simulink model "etherCATmdl3"  (R2022a)
settings: Solver=FixedStepDiscrete  StartTime=0.0  StopTime=inf  RelTol=1e-3
PreLoadFcn:
  | Ts_IO133 = 0.001;
  | Ts_IO750 = 0.001;
InitFcn:
  | Ts_IO133 = 0.001
StopFcn:
  | if isfile(['sdi_view_',bdroot,'.mldatx'])
  |  Simulink.sdi.clearPreferences();
  |  Simulink.sdi.view();
  |  pause(3);
  |  Simulink.sdi.loadView(['sdi_view_',bdroot,]);
  | end
undefined symbols (not defined in the file or in its folder): AUS0, AUS1, C, CAN, FD, padding, Statuswort, Steuerwort
libraries: speedgoatlib_IO602 x9, slrealtimeutilitieslib x8, speedgoatlib_IO133 x5, canfdmsglib x4, canmsglib x4, speedgoatlib_IO750 x4, etargetslib x3, simulink x1
settings Model: SimulationMode=external  ExtModeEnableFloating=off  Creator=sandro.reichenbach  LastModifiedBy=muhammet.cingoez
settings SolverCC: ConcurrentTasks=on  PositivePriorityOrder=on
settings DataIOCC: LimitDataPoints=on  SaveFormat=StructureWithTime
settings OptimizationCC: BlockReduction=off  OptimizeBlockIOStorage=off
settings DebuggingCC: TasksWithSamePriorityMsg=none
settings HardwareCC: ProdBitPerLong=64  ProdLongLongMode=on  ProdHWDeviceType=Intel->x86-64 (Linux 64)
settings RTWCC: Description=Simulink Real-Time  SystemTargetFile=slrealtime.tlc  TemplateMakefile=slrealtime_default_tmf  RTWVerbose=off  Toolchain=Simulink Real-Time Toolchain  BuildConfiguration=Faster Runs  CodeExecutionProfiling=on  TargetLang=C++  DLArmComputeVersion=19.05

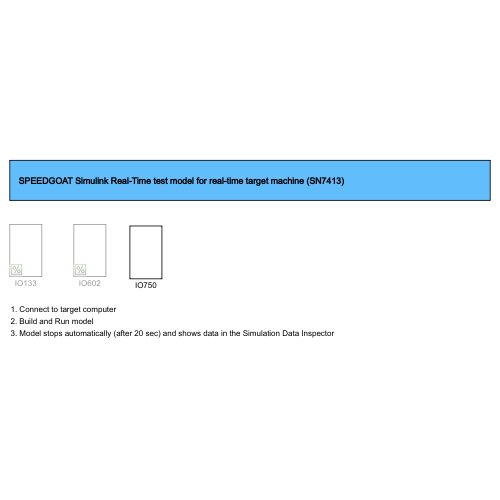
[thumbnail: Simulink's stored preview of the top-level diagram]
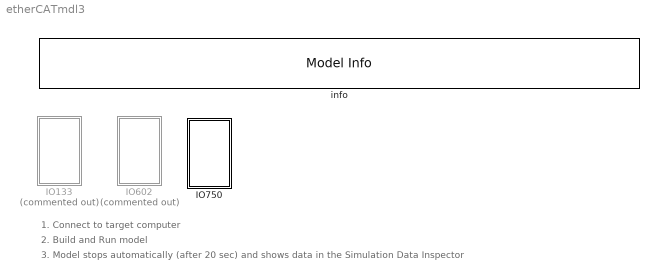
== system etherCATmdl3 ==
  note: 1. Connect to target computer
  note: 2. Build and Run model
  note: 3. Model stops automatically (after 20 sec) and shows data in the Simulation Data Inspector
  IO133 : Subsystem  Commented=on
  IO602 : Subsystem  Commented=on
  IO750 : Subsystem
  info : simulink/Model-Wide Utilities/Model Info  Frame=on  DisplayStringWithTags=SPEEDGOAT Simulink Real-Time test model for real-time target machine (SN7413)  HorizontalTextAlignment=Left  LeftAlignmentValue=0.02

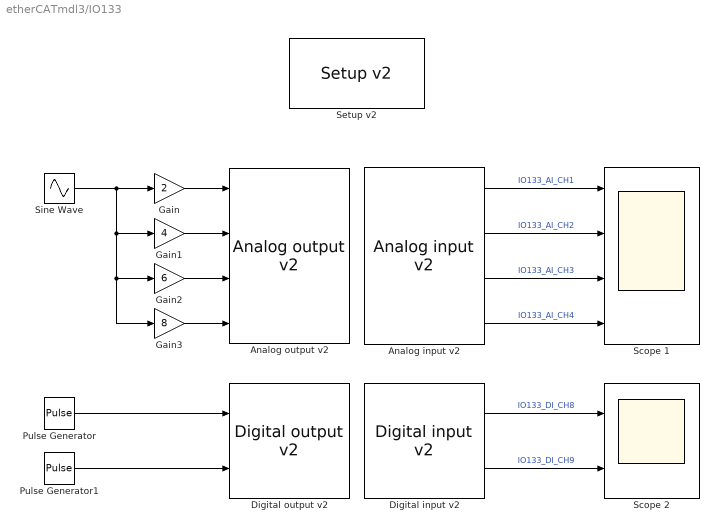
== system etherCATmdl3/IO133 ==
  "Analog input v2 " : speedgoatlib_IO133/Analog input v2   parModuleId=1  parSampleTime=Ts_IO133  parPciSlot=-1  parAdcChannels=[1 2 3 4]  parAdcVoltageRange=[2 2]  parAdcOversamplRate=[1 1]  parAdcContSampling=0  parAdcDmaEnable=0  parAdcActiveDmaDevices=[1 1]  parAdcFrameSize=100
      settings: SourceProductName=Simulink Real-Time: Speedgoat I/O Driver Library
  "Analog output v2 " : speedgoatlib_IO133/Analog output v2   parModuleId=1  parSampleTime=Ts_IO133  parPciSlot=-1  parDacChannels=[1 2 3 4]  parDacVoltageRange=[4 4 6 6 5 5 5 5]  parDacInitValues=[0 0 0 0]  parDacReset=[1 1 1 1]  parDacSyncOut=1  parDacDmaEnable=0  parDacActiveDmaDevices=[1 1]  parDacDmaLatency=2  parDacFrameSize=100
      settings: SourceProductName=Simulink Real-Time: Speedgoat I/O Driver Library
  "Digital input v2 " : speedgoatlib_IO133/Digital input v2   parModuleId=1  parSampleTime=Ts_IO133  parPciSlot=-1  parDiChannels=[8 9]
      settings: SourceProductName=Simulink Real-Time: Speedgoat I/O Driver Library
  "Digital output v2 " : speedgoatlib_IO133/Digital output v2   parModuleId=1  parSampleTime=Ts_IO133  parPciSlot=-1  parDoChannels=[1 2]  parDoInitValues=[0 0]  parDoReset=[1 1]
      settings: SourceProductName=Simulink Real-Time: Speedgoat I/O Driver Library
  Gain : Gain  Gain=2
  Gain1 : Gain  Gain=4
  Gain2 : Gain  Gain=6
  Gain3 : Gain  Gain=8
  Pulse Generator : DiscretePulseGenerator  Period=20  PulseWidth=5  SampleTime=-1
  Pulse Generator1 : DiscretePulseGenerator  Period=20  PulseWidth=10  SampleTime=-1
  Scope 1 : Scope  NumInputPorts=4
  Scope 2 : Scope  NumInputPorts=2
  "Setup v2 " : speedgoatlib_IO133/Setup v2   parPciSlot=-1  parModuleId=1  parInterModuleSync=None  parConvClockBaseRate=20MHz  parConvClock1Divider=20000  parConvClock2Divider=20000  parFrameTriggerEnable=off  parFrameTriggerDivider=10  parConvClock1BaseRate=1  parConvClock2BaseRate=1  parFrameTriggerClock=1  parAdcChannels=1:4  parAdcRange1=+-10V  parAdcRange2=+-10V  parAdcVoltageRange=[2 2]  parAdcOversampling1=None  parAdcOversampling2=None  parAdcOversamplRate=[1 1]  parAdcAutoCorrection=on  parAdcContSampling=off  parAdcDmaEnable=off  parAdcDmaClock=Clock 1  parAdcFrameSize_=100  parAdcSampleTime_=-1  parAdcActiveDmaDevices=[1 1]  parAdcFrameTriggerEnable=0  parAdcFrameSize=100  parAdcSampleTime=0.1  parDacChannels=1:4  parDacInitValues=0  parDacReset=1  parDacRange1=+-5V  parDacRange2=+-5V  parDacRange3=+-10.8V  parDacRange4=+-10.8V  parDacRange5=+-10V  parDacRange6=+-10V  parDacRange7=+-10V  parDacRange8=+-10V  parDacVoltageRange=[4 4 6 6 5 5 5 5]  parDacAutoCorrection=on  parDacSyncOut=on  parDacDmaEnable=off  parDacDmaLatency=Until next frame  parDacDmaClock=Clock 1  parDacFrameSize_=100  parDacSampleTime_=-1  parDacActiveDmaDevices=[1 1]  parDacFrameTriggerEnable=0  parDacFrameSize=100  parDacSampleTime=0.1  parDoChannels=1:2  parDoInitValues=0  parDoReset=1  parDiChannels=8:9  parDiDebounceEnable=off  parDiDebounceTime=0  parDiDebounceValue=0  parDioPullRefFront=Pull-up 3.3V  parDioPullRefRear=Floating
      settings: SourceProductName=Simulink Real-Time: Speedgoat I/O Driver Library
  Sine Wave : Sin  Frequency=50  SampleTime=0
  wires:
  Pulse Generator/1 -> "Digital output v2 "/1
  Gain1/1 -> "Analog output v2 "/2
  Gain/1 -> "Analog output v2 "/1
  Gain3/1 -> "Analog output v2 "/4
  Gain2/1 -> "Analog output v2 "/3
  Sine Wave/1 -> Gain/1, Gain1/1, Gain2/1, Gain3/1
  Pulse Generator1/1 -> "Digital output v2 "/2
  "Analog input v2 "/1 -> Scope 1/1  "IO133_AI_CH1"
  "Analog input v2 "/2 -> Scope 1/2  "IO133_AI_CH2"
  "Analog input v2 "/3 -> Scope 1/3  "IO133_AI_CH3"
  "Analog input v2 "/4 -> Scope 1/4  "IO133_AI_CH4"
  "Digital input v2 "/1 -> Scope 2/1  "IO133_DI_CH8"
  "Digital input v2 "/2 -> Scope 2/2  "IO133_DI_CH9"

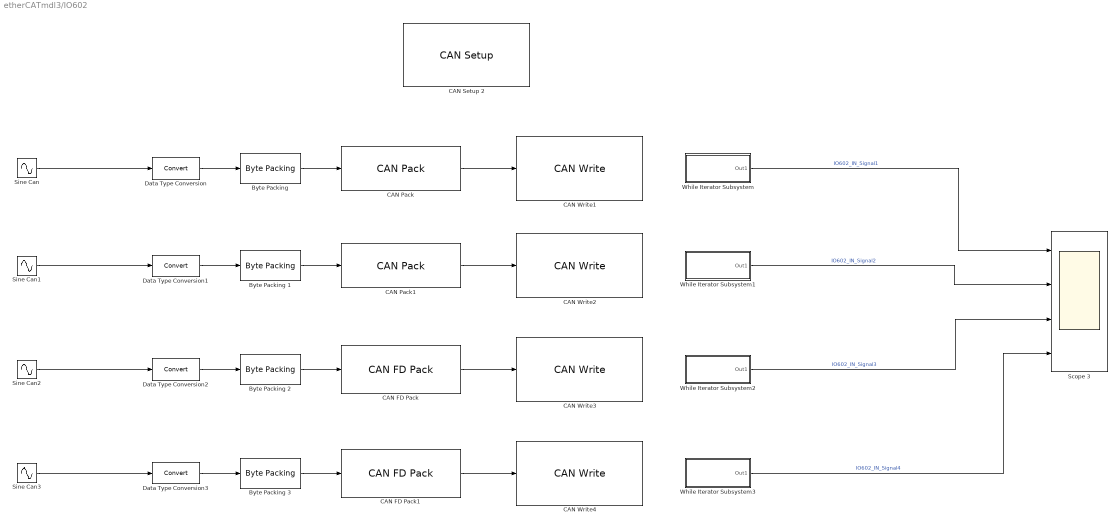
== system etherCATmdl3/IO602 ==
  Byte Packing {,1..3} (4 alike) : slrealtimeutilitieslib/Byte Packing  MaskPackedDataType=uint8  MaskUnpackedDataTypes={'single'}  MaskAlignment=1
  CAN FD Pack : canfdmsglib/CAN FD Pack  MsgList=(none)  MsgName=Msg  ProtocolMode=CAN FD  MsgIDType=Standard (11-bit identifier)  MsgIdentifier=102  MsgLength=4  Remote=off  BRSSwitch=off  ApplyMinMax=off  SignalInfo={}
      settings: SourceProductBaseCode=XP,ME,VN  DataFormat=raw data
  CAN FD Pack1 : canfdmsglib/CAN FD Pack  MsgList=(none)  MsgName=Msg  ProtocolMode=CAN FD  MsgIDType=Standard (11-bit identifier)  MsgIdentifier=103  MsgLength=4  Remote=off  BRSSwitch=off  ApplyMinMax=off  SignalInfo={}
      settings: SourceProductBaseCode=XP,ME,VN  DataFormat=raw data
  CAN Pack : canmsglib/CAN Pack  MsgList=(none)  MsgName=CAN Msg  MsgIDType=Standard (11-bit identifier)  MsgIdentifier=100  MsgLength=4  Remote=off  ApplyMinMax=off  BusOutput=off  SignalInfo={}
      settings: SourceProductBaseCode=XP,ME,VN  DataFormat=raw data
  CAN Pack1 : canmsglib/CAN Pack  MsgList=(none)  MsgName=CAN Msg  MsgIDType=Standard (11-bit identifier)  MsgIdentifier=101  MsgLength=4  Remote=off  ApplyMinMax=off  BusOutput=off  SignalInfo={}
      settings: SourceProductBaseCode=XP,ME,VN  DataFormat=raw data
  CAN Setup 2 : speedgoatlib_IO602/Legacy/CAN Setup   moduletype=IO602  id=1  pciSlot=-1  chn1=CAN (HS)  chn2=CAN (HS)  chn3=CAN-FD  chn4=CAN-FD  initStruct=[]  termStruct=[]  ArbitrationbdrChn1=1.0 MBaud  ArbitrationManbdrChn1=[2,8,31,8]  FdbdrChn1=5.0 MBaud  FdManbdrChn1=[2,2,5,2]  ArbitrationbdrChn2=1.0 MBaud  ArbitrationManbdrChn2=[2,8,31,8]  FdbdrChn2=5.0 MBaud  FdManbdrChn2=[2,2,5,2]  ArbitrationbdrChn3=1.0 MBaud  ArbitrationManbdrChn3=[2,8,31,8]  FdbdrChn3=5.0 MBaud  FdManbdrChn3=[2,2,5,2]  ArbitrationbdrChn4=1.0 MBaud  ArbitrationManbdrChn4=[2,8,31,8]  FdbdrChn4=5.0 MBaud  FdManbdrChn4=[2,2,5,2]  moduleInitValues=[602 1 -1 -1]
      settings: SourceProductName=Simulink Real-Time: Speedgoat I/O Blockset
  CAN Write1 : speedgoatlib_IO602/Legacy/CAN Write  id=1  ts=-1  channel=1  messageType=CAN  BusInput=off  enableStatusPort=off  canType=CAN (HS)  initValues=[602 1 -1 0 1 1 0 0]
      settings: SourceProductName=Simulink Real-Time: Speedgoat I/O Blockset
  CAN Write2 : speedgoatlib_IO602/Legacy/CAN Write  id=1  ts=-1  channel=2  messageType=CAN  BusInput=off  enableStatusPort=off  canType=CAN (HS)  initValues=[602 1 -1 1 1 1 0 0]
      settings: SourceProductName=Simulink Real-Time: Speedgoat I/O Blockset
  CAN Write3 : speedgoatlib_IO602/Legacy/CAN Write  id=1  ts=-1  channel=3  messageType=CAN  BusInput=off  enableStatusPort=off  canType=CAN-FD  initValues=[602 1 -1 2 1 2 0 0]
      settings: SourceProductName=Simulink Real-Time: Speedgoat I/O Blockset
  CAN Write4 : speedgoatlib_IO602/Legacy/CAN Write  id=1  ts=-1  channel=4  messageType=CAN  BusInput=off  enableStatusPort=off  canType=CAN-FD  initValues=[602 1 -1 3 1 2 0 0]
      settings: SourceProductName=Simulink Real-Time: Speedgoat I/O Blockset
  Data Type Conversion{,1..3} (4 alike) : DataTypeConversion  SaturateOnIntegerOverflow=off  RndMeth=Floor
  Scope 3 : Scope  NumInputPorts=4
  Sine Can : Sin  Amplitude=50  Frequency=10*2*pi  SampleTime=0.005
  Sine Can1 : Sin  Amplitude=20  Frequency=10*2*pi  SampleTime=0.005
  Sine Can2 : Sin  Amplitude=30  Frequency=10*2*pi  SampleTime=0.005
  Sine Can3 : Sin  Amplitude=40  Frequency=10*2*pi  SampleTime=0.005
  While Iterator Subsystem : Subsystem  TreatAsAtomicUnit=on
  While Iterator Subsystem1 : Subsystem  TreatAsAtomicUnit=on
  While Iterator Subsystem2 : Subsystem  TreatAsAtomicUnit=on
  While Iterator Subsystem3 : Subsystem  TreatAsAtomicUnit=on
  wires:
  While Iterator Subsystem/1(Out1) -> Scope 3/1  "IO602_IN_Signal1"
  Data Type Conversion/1 -> "Byte Packing "/1
  Sine Can/1 -> Data Type Conversion/1
  CAN Pack/1 -> CAN Write1/1
  "Byte Packing "/1 -> CAN Pack/1
  Byte Packing 1/1 -> CAN Pack1/1
  CAN Pack1/1 -> CAN Write2/1
  Sine Can1/1 -> Data Type Conversion1/1
  Data Type Conversion1/1 -> Byte Packing 1/1
  While Iterator Subsystem1/1(Out1) -> Scope 3/2  "IO602_IN_Signal2"
  While Iterator Subsystem3/1(Out1) -> Scope 3/4  "IO602_IN_Signal4"
  Data Type Conversion3/1 -> Byte Packing 3/1
  Sine Can3/1 -> Data Type Conversion3/1
  CAN FD Pack1/1 -> CAN Write4/1
  Byte Packing 3/1 -> CAN FD Pack1/1
  Byte Packing 2/1 -> CAN FD Pack/1
  CAN FD Pack/1 -> CAN Write3/1
  Sine Can2/1 -> Data Type Conversion2/1
  Data Type Conversion2/1 -> Byte Packing 2/1
  While Iterator Subsystem2/1(Out1) -> Scope 3/3  "IO602_IN_Signal3"

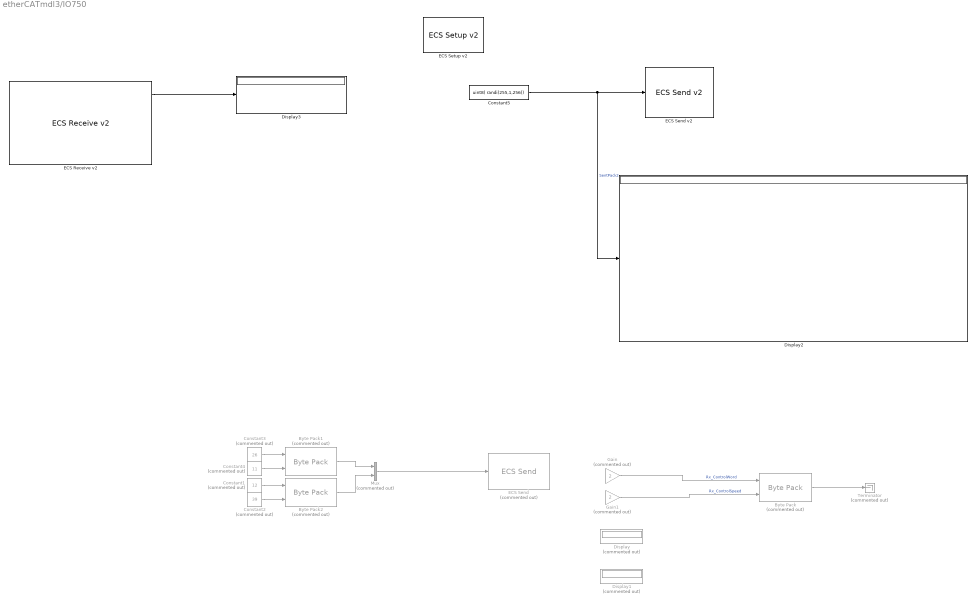
== system etherCATmdl3/IO750 ==
  Byte Pack : etargetslib/Byte Pack  Commented=on  datatypes={'uint32','single'}  byteAlign=1
  Byte Pack1 : etargetslib/Byte Pack  Commented=on  datatypes={'uint32','single'}  byteAlign=1
  Byte Pack2 : etargetslib/Byte Pack  Commented=on  datatypes={'uint32','single'}  byteAlign=1
  Constant1 : Constant  Commented=on  Value=12  OutDataTypeStr=uint32
  Constant2 : Constant  Commented=on  Value=39  OutDataTypeStr=single
  Constant3 : Constant  Commented=on  Value=26  OutDataTypeStr=uint32
  Constant4 : Constant  Commented=on  Value=11  OutDataTypeStr=single
  Constant5 : Constant  Value=uint8( randi(255,1,256))
  Display : Display  Commented=on
  Display1 : Display  Commented=on
  Display2 : Display
  Display3 : Display
  "ECS Receive v2 " : speedgoatlib_IO750/ECS Receive v2   id=1  portType=Separate signals  sampleTime=Ts_IO750  pdoTable={ 'Rx1', 'myvar1', 'single'; 'Rx2', 'myvar2', 'single'; 'Rx3', 'myvar3', 'single' }
      settings: SourceProductName=Simulink Real-Time: Speedgoat I/O Blockset
  ECS Send : speedgoatlib_IO750/ECS Send  Commented=on  id=1  port_type=1 port with n element vector of type UINT8  out_bytes=16  ts=Ts_IO750
      settings: SourceProductName=Simulink Real-Time: Speedgoat I/O Blockset
  "ECS Send v2 " : speedgoatlib_IO750/ECS Send v2   id=1  portType=Byte vector  sampleTime=-1  pdoTable={ 'PDO1', 'myvar1', 'single'; 'PDO2', 'myvar2', 'single'; 'PDO3', 'myvar3', 'single'; 'PDO4', 'myvar4', 'single'; 'PDO5', 'myvar5', 'single'; 'PDO6', 'myvar6', 'single'; 'PDO7', 'myvar7', 'single'; 'PDO8', 'myvar8', 'single'; 'PDO9', 'myvar9', 'single'; 'PDO10', 'myvar10', 'single'; 'PDO11', 'myvar11', 'single'; 'PDO12', 'myvar12', 'single'; 'PDO13', 'myvar13', 'single'; 'PDO14', 'myvar14', 'single'; 'PDO15', 'myvar15', 'single'; 'PDO16', 'myvar16', 'single'; 'PDO17', 'myvar17', 'single'; 'PDO18', 'myvar18', 'single'; 'PDO19', 'myvar19', 'single'; 'PDO20', 'myvar20', 'single'; 'PDO21', 'myvar21', 'single'; 'PDO22', 'myvar22', 'single'; 'PDO23', 'myvar23', 'single'; 'PDO24', 'myvar24', 'single'; 'PDO25', 'myvar25', 'single'; 'PDO26', 'myvar26', 'single'; 'PDO27', 'myvar27', 'single'; 'PDO28', 'myvar28', 'single'; 'PDO29', 'myvar29', 'single'; 'PDO30', 'myvar30', 'single'; 'PDO31', 'myvar31', 'single'; 'PDO32', 'myvar32', 'single'; 'PDO33', 'myvar33', 'single'; 'PDO34', 'myvar34', 'single'; 'PDO35', 'myvar35', 'single'; 'PDO36', 'myvar36', 'single'; 'PDO37', 'myvar37', 'single'; 'PDO38', 'myvar38', 'single'; 'PDO39', 'myvar39', 'single'; 'PDO40', 'myvar40', 'single'; 'PDO41', 'myvar41', 'single'; 'PDO42', 'myvar42', 'single'; 'PDO43', 'myvar43', 'single'; 'PDO44', 'myvar44', 'single'; 'PDO45', 'myvar45', 'single'; 'PDO46', 'myvar46', 'single'; 'PDO47', 'myvar47', 'single'; 'PDO48', 'myvar48', 'single'; 'PDO49', 'myvar49', 'single'; 'PDO50', 'myvar50', 'single'; 'PDO51', 'myvar51', 'single'; 'PDO52', 'myvar52', 'single'; 'PDO53', 'myvar53', 'single'; 'PDO54', 'myvar54', 'single'; 'PDO55', 'myvar55', 'single'; 'PDO56', 'myvar56', 'single'; 'PDO57', 'myvar57', 'single'; 'PDO58', 'myvar58', 'single'; 'PDO59', 'myvar59', 'single'; 'PDO60', 'myvar60', 'single'; 'PDO61', 'myvar61', 'single'; 'PDO62', 'myvar62', 'single'; 'PDO63', 'myvar63', 'single'; 'PDO64', 'myvar64', 'single' }
      settings: SourceProductName=Simulink Real-Time: Speedgoat I/O Blockset
  "ECS Setup v2 " : speedgoatlib_IO750/ECS Setup v2   id=1  drvLetter=C:  configurationMode=Warmstart  busSlot=-1  busStartup=Automatic  dcSync=off  vendorName='Speedgoat'  groupName='Automation'  typeName='IO750'  vendorID=hex2dec('00000001')  productCode=hex2dec('00000002')  revisionNo=hex2dec('00000003')  serialNo=hex2dec('00000004')  stationAlias=0  deviceIdent=0  rxPdoMapping={ 'Rx1', 'myvar1', 'single'; 'Rx2', 'myvar2', 'single'; 'Rx3', 'myvar3', 'single' }  rxPdoCfg=0  rxPdoNames=,Steuerwort,Steuerwort,Statuswort  rxVarNames=,AUS0,padding,AUS1  txPdoMapping={ 'PDO1', 'myvar1', 'single'; 'PDO2', 'myvar2', 'single'; 'PDO3', 'myvar3', 'single'; 'PDO4', 'myvar4', 'single'; 'PDO5', 'myvar5', 'single'; 'PDO6', 'myvar6', 'single'; 'PDO7', 'myvar7', 'single'; 'PDO8', 'myvar8', 'single'; 'PDO9', 'myvar9', 'single'; 'PDO10', 'myvar10', 'single'; 'PDO11', 'myvar11', 'single'; 'PDO12', 'myvar12', 'single'; 'PDO13', 'myvar13', 'single'; 'PDO14', 'myvar14', 'single'; 'PDO15', 'myvar15', 'single'; 'PDO16', 'myvar16', 'single'; 'PDO17', 'myvar17', 'single'; 'PDO18', 'myvar18', 'single'; 'PDO19', 'myvar19', 'single'; 'PDO20', 'myvar20', 'single'; 'PDO21', 'myvar21', 'single'; 'PDO22', 'myvar22', 'single'; 'PDO23', 'myvar23', 'single'; 'PDO24', 'myvar24', 'single'; 'PDO25', 'myvar25', 'single'; 'PDO26', 'myvar26', 'single'; 'PDO27', 'myvar27', 'single'; 'PDO28', 'myvar28', 'single'; 'PDO29', 'myvar29', 'single'; 'PDO30', 'myvar30', 'single'; 'PDO31', 'myvar31', 'single'; 'PDO32', 'myvar32', 'single'; 'PDO33', 'myvar33', 'single'; 'PDO34', 'myvar34', 'single'; 'PDO35', 'myvar35', 'single'; 'PDO36', 'myvar36', 'single'; 'PDO37', 'myvar37', 'single'; 'PDO38', 'myvar38', 'single'; 'PDO39', 'myvar39', 'single'; 'PDO40', 'myvar40', 'single'; 'PDO41', 'myvar41', 'single'; 'PDO42', 'myvar42', 'single'; 'PDO43', 'myvar43', 'single'; 'PDO44', 'myvar44', 'single'; 'PDO45', 'myvar45', 'single'; 'PDO46', 'myvar46', 'single'; 'PDO47', 'myvar47', 'single'; 'PDO48', 'myvar48', 'single'; 'PDO49', 'myvar49', 'single'; 'PDO50', 'myvar50', 'single'; 'PDO51', 'myvar51', 'single'; 'PDO52', 'myvar52', 'single'; 'PDO53', 'myvar53', 'single'; 'PDO54', 'myvar54', 'single'; 'PDO55', 'myvar55', 'single'; 'PDO56', 'myvar56', 'single'; 'PDO57', 'myvar57', 'single'; 'PDO58', 'myvar58', 'single'; 'PDO59', 'myvar59', 'single'; 'PDO60', 'myvar60', 'single'; 'PDO61', 'myvar61', 'single'; 'PDO62', 'myvar62', 'single'; 'PDO63', 'myvar63', 'single'; 'PDO64', 'myvar64', 'single' }  txPdoCfg=0  txPdoNames=0  txVarNames=0  sdoMapping={}  sdoCfg=0  sdoNames=0  qtyMods=[1,0,0]  moduleType=IO750  protocol=IO750  firmware=EtherCAT Slave
      settings: SourceProductName=Simulink Real-Time: Speedgoat I/O Blockset
  Gain : Gain  Commented=on  Gain=2  OutDataTypeStr=uint32
  Gain1 : Gain  Commented=on  Gain=2
  Mux : Mux  Commented=on  Inputs=2
  Terminator : Terminator  Commented=on
  wires:
  ? -> Display1/1, Gain1/1
  ? -> Display/1, Gain/1
  Constant3/1 -> Byte Pack1/1
  Constant4/1 -> Byte Pack1/2
  Gain1/1 -> Byte Pack/2  "Rx_ControlSpeed"
  Gain/1 -> Byte Pack/1  "Rx_ControlWord"
  Mux/1 -> ECS Send/1
  Byte Pack1/1 -> Mux/1
  Constant2/1 -> Byte Pack2/2
  Constant1/1 -> Byte Pack2/1
  Byte Pack2/1 -> Mux/2
  Byte Pack/1 -> Terminator/1
  Constant5/1 -> Display2/1, "ECS Send v2 "/1  "SentPack2"
  "ECS Receive v2 "/1 -> Display3/1

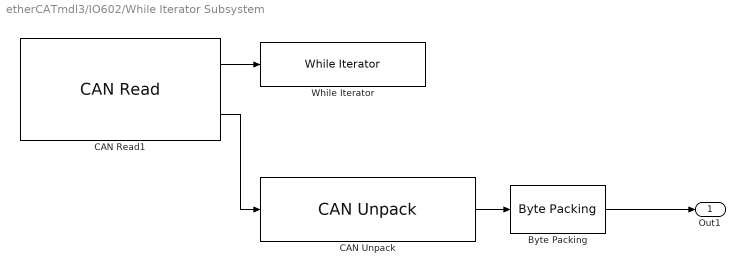
== system etherCATmdl3/IO602/While Iterator Subsystem ==
  "Byte Packing " : slrealtimeutilitieslib/Byte Packing  MaskPackedDataType=single  MaskUnpackedDataTypes={'uint8'}  MaskAlignment=1
  CAN Read1 : speedgoatlib_IO602/Legacy/CAN Read  id=1  ts=-1  channel=1  messageType=CAN  canType=CAN (HS)  BusOutput=off  initValues=[602 1 -1 0 1 1 0]
      settings: SourceProductName=Simulink Real-Time: Speedgoat I/O Blockset
  CAN Unpack : canmsglib/CAN Unpack  MsgList=(none)  MsgName=CAN Msg  MsgIDType=Standard (11-bit identifier)  MsgIdentifier=101  MsgLength=4  SignalInfo={}  IDPort=off  TimestampPort=off  ErrorPort=off  RemotePort=off  LengthPort=off  StatusPort=off  ApplyMinMax=off
      settings: SourceProductBaseCode=XP,ME,VN  DataFormat=raw data
  While Iterator : WhileIterator  MaxIters=50  WhileBlockType=do-while
  Out1 : Outport
  wires:
  "Byte Packing "/1 -> Out1/1
  CAN Unpack/1 -> "Byte Packing "/1
  CAN Read1/2 -> CAN Unpack/1
  CAN Read1/1 -> While Iterator/1

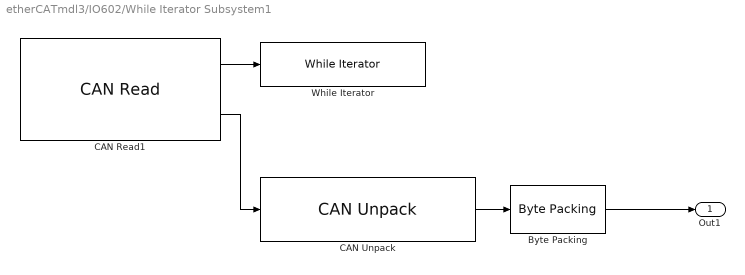
== system etherCATmdl3/IO602/While Iterator Subsystem1 ==
  "Byte Packing " : slrealtimeutilitieslib/Byte Packing  MaskPackedDataType=single  MaskUnpackedDataTypes={'uint8'}  MaskAlignment=1
  CAN Read1 : speedgoatlib_IO602/Legacy/CAN Read  id=1  ts=-1  channel=2  messageType=CAN  canType=CAN (HS)  BusOutput=off  initValues=[602 1 -1 1 1 1 0]
      settings: SourceProductName=Simulink Real-Time: Speedgoat I/O Blockset
  CAN Unpack : canmsglib/CAN Unpack  MsgList=(none)  MsgName=CAN Msg  MsgIDType=Standard (11-bit identifier)  MsgIdentifier=100  MsgLength=4  SignalInfo={}  IDPort=off  TimestampPort=off  ErrorPort=off  RemotePort=off  LengthPort=off  StatusPort=off  ApplyMinMax=off
      settings: SourceProductBaseCode=XP,ME,VN  DataFormat=raw data
  While Iterator : WhileIterator  MaxIters=50  WhileBlockType=do-while
  Out1 : Outport
  wires:
  CAN Read1/1 -> While Iterator/1
  CAN Read1/2 -> CAN Unpack/1
  CAN Unpack/1 -> "Byte Packing "/1
  "Byte Packing "/1 -> Out1/1

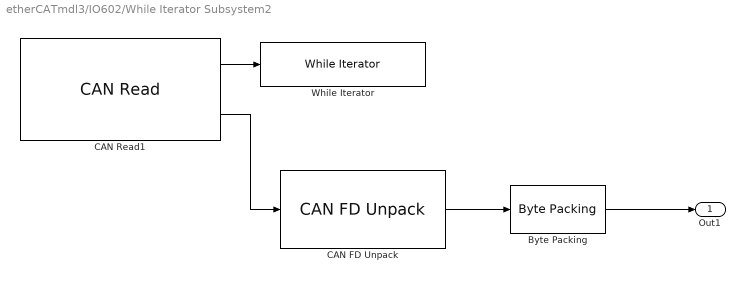
== system etherCATmdl3/IO602/While Iterator Subsystem2 ==
  "Byte Packing " : slrealtimeutilitieslib/Byte Packing  MaskPackedDataType=single  MaskUnpackedDataTypes={'uint8'}  MaskAlignment=1
  CAN FD Unpack : canfdmsglib/CAN FD Unpack  MsgList=(none)  MsgName=Msg  ProtocolMode=CAN FD  MsgIDType=Standard (11-bit identifier)  MsgIdentifier=103  MsgLength=4  SignalInfo={}  IDPort=off  TimestampPort=off  ErrorPort=off  RemotePort=off  LengthPort=off  StatusPort=off  BRSPort=off  ESIPort=off  DLCPort=off  ApplyMinMax=off
      settings: SourceProductBaseCode=XP,ME,VN  DataFormat=raw data
  CAN Read1 : speedgoatlib_IO602/Legacy/CAN Read  id=1  ts=-1  channel=3  messageType=CAN  canType=CAN-FD  BusOutput=off  initValues=[602 1 -1 2 1 2 0]
      settings: SourceProductName=Simulink Real-Time: Speedgoat I/O Blockset
  While Iterator : WhileIterator  MaxIters=50  WhileBlockType=do-while
  Out1 : Outport
  wires:
  CAN Read1/1 -> While Iterator/1
  CAN Read1/2 -> CAN FD Unpack/1
  CAN FD Unpack/1 -> "Byte Packing "/1
  "Byte Packing "/1 -> Out1/1

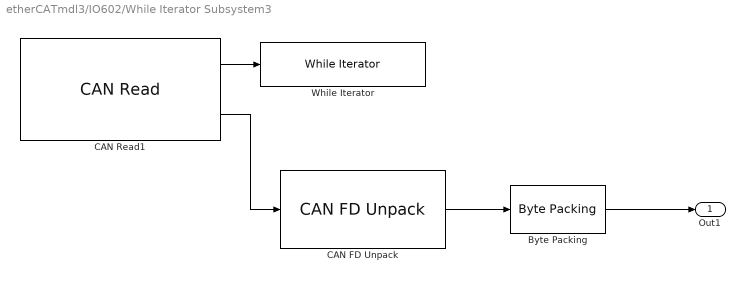
== system etherCATmdl3/IO602/While Iterator Subsystem3 ==
  "Byte Packing " : slrealtimeutilitieslib/Byte Packing  MaskPackedDataType=single  MaskUnpackedDataTypes={'uint8'}  MaskAlignment=1
  CAN FD Unpack : canfdmsglib/CAN FD Unpack  MsgList=(none)  MsgName=Msg  ProtocolMode=CAN FD  MsgIDType=Standard (11-bit identifier)  MsgIdentifier=102  MsgLength=4  SignalInfo={}  IDPort=off  TimestampPort=off  ErrorPort=off  RemotePort=off  LengthPort=off  StatusPort=off  BRSPort=off  ESIPort=off  DLCPort=off  ApplyMinMax=off
      settings: SourceProductBaseCode=XP,ME,VN  DataFormat=raw data
  CAN Read1 : speedgoatlib_IO602/Legacy/CAN Read  id=1  ts=-1  channel=4  messageType=CAN  canType=CAN-FD  BusOutput=off  initValues=[602 1 -1 3 1 2 0]
      settings: SourceProductName=Simulink Real-Time: Speedgoat I/O Blockset
  While Iterator : WhileIterator  MaxIters=50  WhileBlockType=do-while
  Out1 : Outport
  wires:
  "Byte Packing "/1 -> Out1/1
  CAN FD Unpack/1 -> "Byte Packing "/1
  CAN Read1/2 -> CAN FD Unpack/1
  CAN Read1/1 -> While Iterator/1
